simulink model "CompControl"  (R2025b)
settings: Solver=VariableStepAuto  StartTime=0.0  StopTime=10.0  RelTol=1e-3
values from neighbouring files (symbols this model uses):
  K_d = 40    [NewRun.m]
  K_p = 400    [NewRun.m]
settings Model: Creator=ironc  LastModifiedBy=ironc

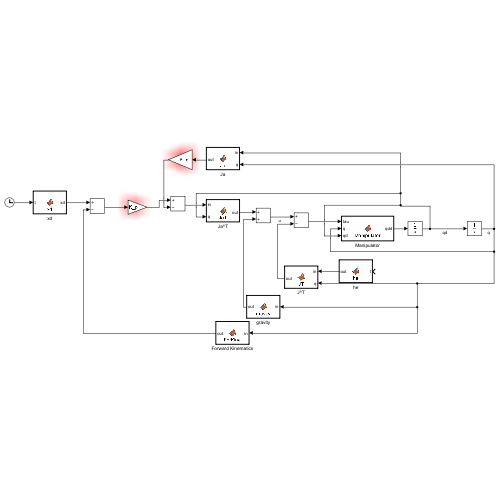
[thumbnail: Simulink's stored preview of the top-level diagram]
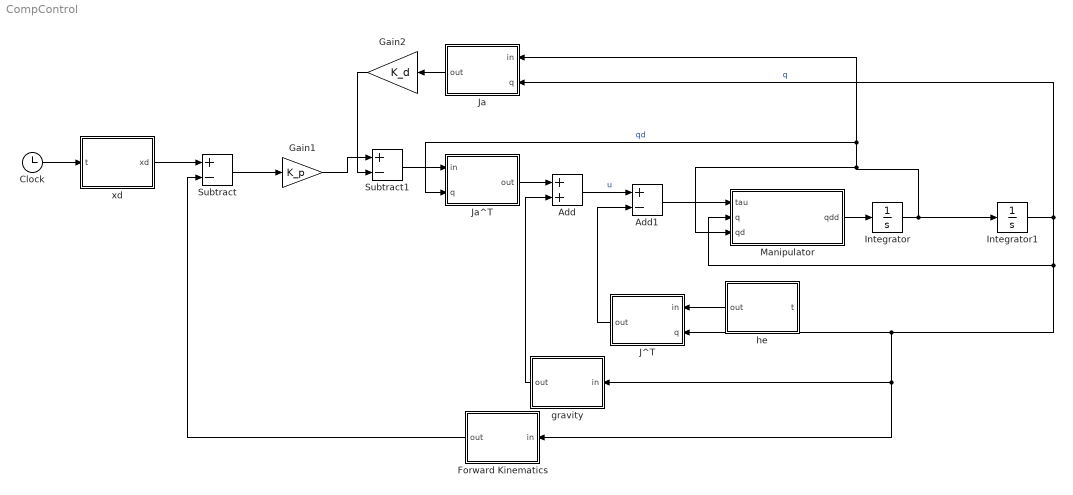
== system CompControl ==
  Add : Sum
  Add1 : Sum  Inputs=+-
  Clock : Clock
  Forward Kinematics : MATLAB Function  TreatAsAtomicUnit=on
  Gain1 : Gain  Gain=K_p
  Gain2 : Gain  Gain=K_d
  Integrator : Integrator
  Integrator1 : Integrator
  J^T : MATLAB Function  TreatAsAtomicUnit=on
  Ja : MATLAB Function  TreatAsAtomicUnit=on
  Ja^T : MATLAB Function  TreatAsAtomicUnit=on
  Manipulator : MATLAB Function  TreatAsAtomicUnit=on
  Subtract : Sum  Inputs=+-
  Subtract1 : Sum  Inputs=+-
  gravity : MATLAB Function  TreatAsAtomicUnit=on
  he : MATLAB Function  TreatAsAtomicUnit=on
  xd : MATLAB Function  TreatAsAtomicUnit=on
  wires:
  xd/1(xd) -> Subtract/1
  Subtract/1 -> Gain1/1
  Gain1/1 -> Subtract1/1
  Subtract1/1 -> Ja^T/1(in)
  Gain2/1 -> Subtract1/2
  Ja/1(out) -> Gain2/1
  Ja^T/1(out) -> Add/1
  Add/1 -> Add1/1  "u"
  Add1/1 -> Manipulator/1(tau)
  Integrator/1 -> Integrator1/1, Manipulator/3(qd), Ja^T/2(q), Ja/1(in)  "qd"
  Integrator1/1 -> Ja/2(q), Manipulator/2(q), J^T/2(q), Forward Kinematics/1(in), gravity/1(in)  "q"
  gravity/1(out) -> Add/2
  J^T/1(out) -> Add1/2
  Forward Kinematics/1(out) -> Subtract/2
  he/1(out) -> J^T/1(in)
  Manipulator/1(qdd) -> Integrator/1
  Clock/1 -> xd/1(t)

== matlab function CompControl/Ja ==
  data: out output; in input; q input
function out = Ja(in,q)

out = in;

== matlab function CompControl/Ja^T ==
  data: in input; out output; q input
function out = JaT(in,q)

out = in;

== matlab function CompControl/Manipulator ==
  data: tau input; q input; qd input; qdd output
function qdd = Manipulator(tau,q,qd)



end

== matlab function CompControl/gravity ==
  data: in input; out output
function out = gravity(in)

out = in;

== matlab function CompControl/J^T ==
  data: in input; out output; q input
function out = JT(in,q)

out = in;

== matlab function CompControl/Forward Kinematics ==
  data: in input; out output
function out = ForKine(in)

out = in;

== matlab function CompControl/he ==
  data: t input; out output
function out = he(t)

out = t;

== matlab function CompControl/xd ==
  data: t input; xd output
function xd = xd(t)

xd = t;
